simulink model "CompleteAttDetSim"  (R2019b)
settings: Solver=FixedStepAuto  StartTime=0.0  StopTime=24*3600  FixedStep=10  RelTol=1e-3  EnableMultiTasking=on
PreLoadFcn:
  | InitialiseJ2
undefined symbols (not defined in the file): a, e, Earth, h, i, J2, mu, omega, R_earth, RAAN, T, t0, WGS84
libraries: vrlib x11, sharedtransform x9, aerolibutil x5, dspindex x1, aerolibtransform2 x1
settings Model: PauseTimes=0  NumberOfSteps=10  SnapshotBufferSize=10000  SnapshotInterval=1  Creator="TEAM  STUDSAT -2"  LastModifiedBy=zackm
settings DataIOCC: ReturnWorkspaceOutputs=off
settings OptimizationCC: LifeSpan=inf
settings DebuggingCC: SFUnexpectedBacktrackingDiag=warning  SFNoUnconditionalDefaultTransitionDiag=warning  SFExecutionAtInitializationDiag=none  ArithmeticOperatorsInVariantConditions=warning
settings SFSimCC: SimUseLocalCustomCode=off  CustomCodeUndefinedFunction=UseInterfaceOnly
settings RTWCC: RTWUseLocalCustomCode=off
settings CodeAppCC: StateflowObjectComments=on
settings GRTTargetCC: TargetLangStandard=C89/C90 (ANSI)  GeneratePreprocessorConditionals=Disable all
settings ConfigComp: CovMetricSettings=dw  CovHtmlReporting=on  CovSaveCumulativeToWorkspaceVar=on  CovSaveSingleToWorkspaceVar=on  CovExternalEMLEnable=off

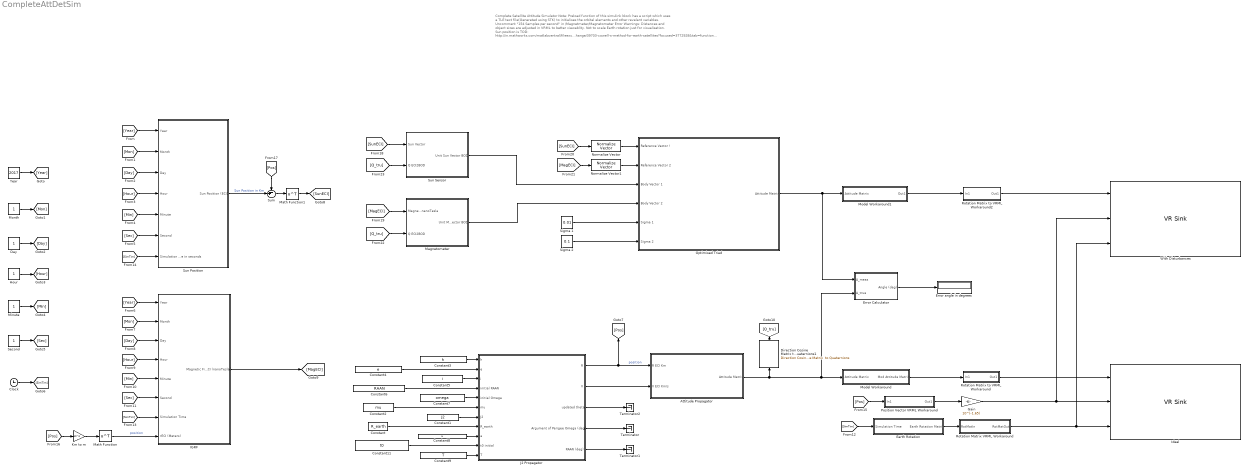
== system CompleteAttDetSim ==
  note: Complete Satellite Attitude Simulator
      |
      | Note:
      | Preload function of this simulink block has a script which uses a TLE text file(Generated using STK) to initialises the orbital elements and other revelant variables.
      | Uncomment "154 Samples per second" in /Magnetmeter/Magnetometer Error
      |
      | Warnings:
      | Distances and object sizes are adjusted in VRML to better viewablity. Not to scale
      | Earth rotation just for visualisation.
      | Sun position is TOD: http://in.mathworks.com/matlabcentral/fileexchange/39703-cowell-s-method-for-earth-satellites?focused=3772928&tab=function
      | Magnetometer model needs improvements
  " Magnetometer" : Subsystem
  " Sun Position" : Subsystem
  Attitude Propagator : Subsystem
  Clock : Clock
  Constant : Constant  Value=R_earth
  Constant1 : Constant  Value=J2
  Constant11 : Constant  Value=t0
  Constant2 : Constant  Value=mu
  Constant3 : Constant  Value=h
  Constant4 : Constant  Value=e
  Constant5 : Constant  Value=i
  Constant6 : Constant  Value=RAAN
  Constant7 : Constant  Value=omega
  Constant8 : Constant  Value=a
  Constant9 : Constant  Value=T
  Day : Constant
  Direction Cosine Matrix to Quaternions1 : sharedtransform/Direction Cosine Matrix  to Quaternions  aMode=aMode  action=None  tolerance=eps(2)
      settings: SourceProductName=Aerospace Blockset  SourceProductBaseCode=AE
  Earth Rotation : Subsystem
  Error Calculator : Subsystem
  Error angle in degrees : Display
  Gain : Gain  Gain=10^(-1.65)
  Hour : Constant
  IGRF : Subsystem
  Ideal : vrlib/VR Sink  InstantiateOnLoad=on  SampleTime=-1  ViewEnable=on  RemoteChange=off  RemoteView=off  FieldsWritten=Satellite.rotation.4.1.1.double#Satellite.translation.3.1.1.double#Earth.rotation.4.1.1.double  WorldFileName=earthSatSys_Ideal.WRL  AutoView=off  VideoDimensions=[]  AllowVariableSize=off
      settings: SourceProductBaseCode=VR
  J2 Propagator : Subsystem
  Km to m : Gain  Gain=10^3
  Math Function : Math  Operator=transpose  SaturateOnIntegerOverflow=on
  Math Function1 : Math  Operator=transpose  SaturateOnIntegerOverflow=on
  Minute : Constant
  Model Workaround : Subsystem
  Model Workaround1 : Subsystem
  Month : Constant
  Normalize Vector : vrlib/Utilities/Normalize Vector  maxzero=0
      settings: SourceProductName=Simulink 3D Animation  SourceProductBaseCode=VR
  Normalize Vector1 : vrlib/Utilities/Normalize Vector  maxzero=0
      settings: SourceProductName=Simulink 3D Animation  SourceProductBaseCode=VR
  Optimised Triad : Subsystem
  Position Vector VRML Workaround : Subsystem
  Rotation Matrix VRML Workaround : Subsystem
  Rotation Matrix to VRML Workaround : Subsystem
  Rotation Matrix to VRML Workaround2 : Subsystem
  Second : Constant
  Sigma 1 : Constant  Value=0.01
  Sigma 2 : Constant  Value=0.1
  Sum : Sum  Inputs=-+|
  Sun Sensor : Subsystem
  Terminator : Terminator
  Terminator1 : Terminator
  Terminator2 : Terminator
  With Disturbances : vrlib/VR Sink  InstantiateOnLoad=on  SampleTime=-1  ViewEnable=on  RemoteChange=off  RemoteView=off  FieldsWritten=Satellite1.rotation.4.1.1.double#Satellite1.translation.3.1.1.double#Earth1.rotation.4.1.1.double  WorldFileName=earthSatSys_Real.WRL  AutoView=off  VideoDimensions=[]  AllowVariableSize=off
      settings: SourceProductBaseCode=VR
  Year : Constant  Value=2017
  wires:
  Constant/1 -> J2 Propagator/8(R_earth)
  Constant1/1 -> J2 Propagator/7(J2)
  Constant2/1 -> J2 Propagator/6(mu)
  Constant3/1 -> J2 Propagator/1(h)
  Constant4/1 -> J2 Propagator/2(e)
  Constant5/1 -> J2 Propagator/3(i)
  Constant6/1 -> J2 Propagator/4(initial RAAN)
  Constant8/1 -> J2 Propagator/9(a)
  Constant11/1 -> J2 Propagator/10(t0 initial)
  Constant9/1 -> J2 Propagator/11(T)
  Constant7/1 -> J2 Propagator/5(initial Omega)
  J2 Propagator/4(Argument of Perigee Omega (deg)) -> Terminator/1
  Earth Rotation/1(Earth Rotation Matrix) -> Rotation Matrix VRML Workaround/1(RotMatIn)
  Position Vector VRML Workaround/1(Out1) -> Gain/1
  J2 Propagator/5(RAAN (deg)) -> Terminator1/1
  Gain/1 -> With Disturbances/2, Ideal/2
  Rotation Matrix VRML Workaround/1(RotMatOut) -> With Disturbances/3, Ideal/3
  J2 Propagator/3(updated theta) -> Terminator2/1
  Model Workaround/1(Mod Attitude Matrix) -> Rotation Matrix to VRML Workaround/1(In1)
  J2 Propagator/2(V) -> Attitude Propagator/2(V ECI Km/s)
  Rotation Matrix to VRML Workaround/1(Out1) -> Ideal/1
  Model Workaround1/1(Out1) -> Rotation Matrix to VRML Workaround2/1(In1)
  Sigma 2/1 -> Optimised Triad/6(Sigma 2)
  Optimised Triad/1(Attitude Matrix) -> Error Calculator/1(A_meas), Model Workaround1/1(Attitude Matrix)
  Rotation Matrix to VRML Workaround2/1(Out1) -> With Disturbances/1
  Sigma 1/1 -> Optimised Triad/5(Sigma 1)
  " Magnetometer"/1(Unit Magnetic Field Vector BOD) -> Optimised Triad/4(Body Vector 2)
  Error Calculator/1(Angle (deg)) -> Error angle in degrees/1
  Km to m/1 -> Math Function/1
  " Sun Position"/1(Sun Position (ECI)) -> Sum/2  "Sun Position in Km"
  Attitude Propagator/1(Attitude Matrix) -> Direction Cosine Matrix to Quaternions1/1, Error Calculator/2(A_true), Model Workaround/1(Attitude Matrix)
  Sun Sensor/1(Unit Sun Vector BOD) -> Optimised Triad/3(Body Vector 1)
  Year/1 -> [Year]
  Month/1 -> [Mon]
  Day/1 -> [Day]
  Hour/1 -> [Hour]
  Minute/1 -> [Min]
  Second/1 -> [Sec]
  [Year] -> " Sun Position"/1(Year)
  [Mon] -> " Sun Position"/2("Month ")
  [Day] -> " Sun Position"/3(Day)
  [Hour] -> " Sun Position"/4(Hour)
  [Min] -> " Sun Position"/5(Minute)
  [Sec] -> " Sun Position"/6(Second)
  [Year] -> IGRF/1(Year)
  [Mon] -> IGRF/2(Month)
  [Day] -> IGRF/3(Day)
  [Hour] -> IGRF/4(Hour)
  [Min] -> IGRF/5(Minute)
  [Sec] -> IGRF/6(Second)
  Clock/1 -> [SimTim]
  [SimTim] -> Earth Rotation/1(Simulation Time)
  [SimTim] -> IGRF/7(Simulation Time)
  [SimTim] -> " Sun Position"/7(" Simulation time in seconds")
  J2 Propagator/1(R) -> [Pos], Attitude Propagator/1(R ECI Km)  "position"
  [Pos] -> Position Vector VRML Workaround/1(In1)
  [Pos] -> Km to m/1
  Math Function/1 -> IGRF/8(rECI (Meters))  "position"
  [Pos] -> Sum/1
  Sum/1 -> Math Function1/1
  IGRF/1(Magnetic Field in ECI (nanoTesla)) -> [MagECI]
  [SunECI] -> Sun Sensor/1(Sun Vector)
  [MagECI] -> " Magnetometer"/1(Magnettic Field ECI nanoTesla)
  [SunECI] -> Normalize Vector/1
  [MagECI] -> Normalize Vector1/1
  Normalize Vector/1 -> Optimised Triad/1(Reference Vector !)
  Normalize Vector1/1 -> Optimised Triad/2(Reference Vector 2)
  Direction Cosine Matrix to Quaternions1/1 -> [Q_tru]
  [Q_tru] -> " Magnetometer"/2(Q ECI2BOD)
  [Q_tru] -> Sun Sensor/2(Q ECI2BOD)
  Math Function1/1 -> [SunECI]

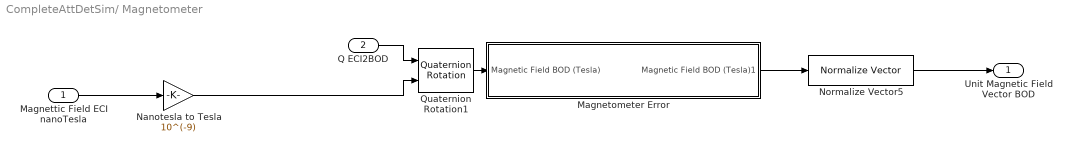
== system CompleteAttDetSim/ Magnetometer ==
  Magnettic Field ECI nanoTesla : Inport
  Q ECI2BOD : Inport  Port=2
  Magnetometer Error : Subsystem
  Nanotesla to Tesla : Gain  Gain=10^(-9)
  Normalize Vector5 : vrlib/Utilities/Normalize Vector  maxzero=0
      settings: SourceProductName=Simulink 3D Animation  SourceProductBaseCode=VR
  Quaternion Rotation1 : aerolibutil/Quaternion Rotation
  Unit Magnetic Field Vector BOD : Outport
  wires:
  Magnettic Field ECI nanoTesla/1 -> Nanotesla to Tesla/1
  Magnetometer Error/1("Magnetic Field BOD (Tesla)1 ") -> Normalize Vector5/1
  Normalize Vector5/1 -> Unit Magnetic Field Vector BOD/1
  Q ECI2BOD/1 -> Quaternion Rotation1/1
  Nanotesla to Tesla/1 -> Quaternion Rotation1/2
  Quaternion Rotation1/1 -> Magnetometer Error/1(Magnetic Field BOD (Tesla))

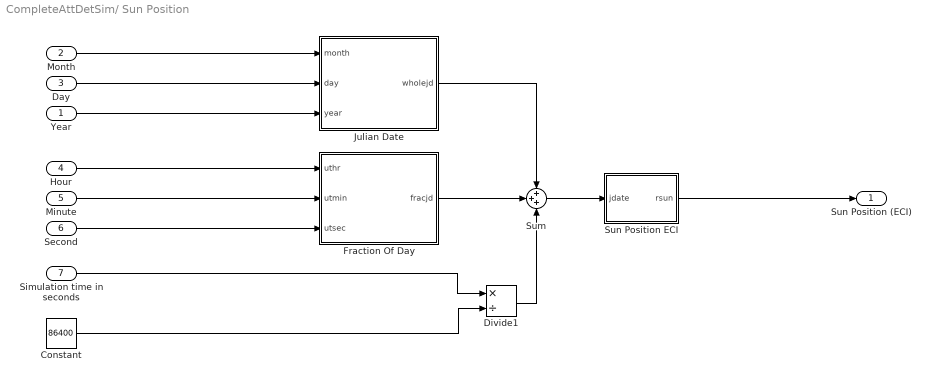
== system CompleteAttDetSim/ Sun Position ==
  Year : Inport
  "Month " : Inport  Port=2
  Day : Inport  Port=3
  Hour : Inport  Port=4
  Minute : Inport  Port=5
  Second : Inport  Port=6
  " Simulation time in seconds" : Inport  Port=7
  Constant : Constant  Value=86400
  Divide1 : Product  Inputs=*/
  Fraction Of Day : MATLAB Function  TreatAsAtomicUnit=on
  Julian Date : MATLAB Function  TreatAsAtomicUnit=on
  Sum : Sum  Inputs=+++
  Sun Position ECI : MATLAB Function  TreatAsAtomicUnit=on
  Sun Position (ECI) : Outport
  wires:
  Sum/1 -> Sun Position ECI/1(jdate)
  " Simulation time in seconds"/1 -> Divide1/1
  Sun Position ECI/1(rsun) -> Sun Position (ECI)/1
  Second/1 -> Fraction Of Day/3(utsec)
  Fraction Of Day/1(fracjd) -> Sum/2
  Year/1 -> Julian Date/3(year)
  Day/1 -> Julian Date/2(day)
  Divide1/1 -> Sum/3
  Minute/1 -> Fraction Of Day/2(utmin)
  Julian Date/1(wholejd) -> Sum/1
  Constant/1 -> Divide1/2
  Hour/1 -> Fraction Of Day/1(uthr)
  "Month "/1 -> Julian Date/1(month)

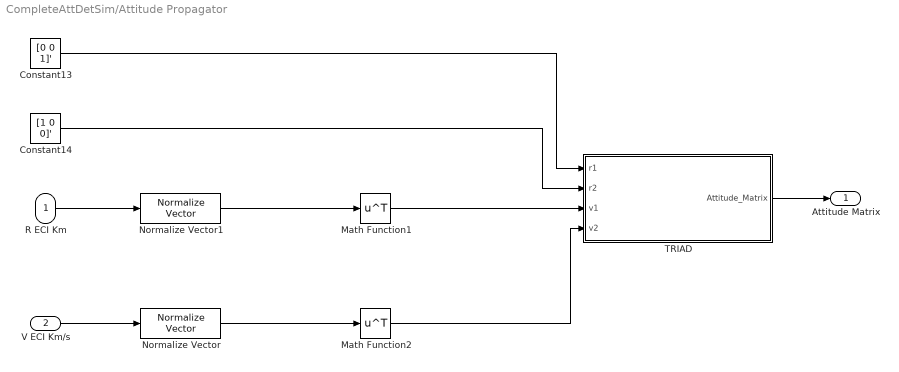
== system CompleteAttDetSim/Attitude Propagator ==
  R ECI Km : Inport
  V ECI Km/s : Inport  Port=2
  Constant13 : Constant  Value=[0 0 1]'  VectorParams1D=off
  Constant14 : Constant  Value=[1 0 0]'  VectorParams1D=off
  Math Function1 : Math  Operator=transpose  SaturateOnIntegerOverflow=on
  Math Function2 : Math  Operator=transpose  SaturateOnIntegerOverflow=on
  Normalize Vector : vrlib/Utilities/Normalize Vector  maxzero=0
      settings: SourceProductName=Simulink 3D Animation  SourceProductBaseCode=VR
  Normalize Vector1 : vrlib/Utilities/Normalize Vector  maxzero=0
      settings: SourceProductName=Simulink 3D Animation  SourceProductBaseCode=VR
  TRIAD : MATLAB Function  TreatAsAtomicUnit=on
  Attitude Matrix : Outport
  wires:
  Constant13/1 -> TRIAD/1(r1)
  TRIAD/1(Attitude_Matrix) -> Attitude Matrix/1
  Math Function1/1 -> TRIAD/3(v1)
  Math Function2/1 -> TRIAD/4(v2)
  Constant14/1 -> TRIAD/2(r2)
  V ECI Km/s/1 -> Normalize Vector/1
  Normalize Vector/1 -> Math Function2/1
  Normalize Vector1/1 -> Math Function1/1
  R ECI Km/1 -> Normalize Vector1/1

== system CompleteAttDetSim/Earth Rotation ==
  Simulation Time : Inport
  Constant10 : Constant  Value=0.004178074378280
  Subsystem1 : Subsystem
  Earth Rotation Matrix : Outport
  wires:
  Constant10/1 -> Subsystem1/1(we)
  Simulation Time/1 -> Subsystem1/2(Clock)
  Subsystem1/1(Earth Rotation Matrix) -> Earth Rotation Matrix/1

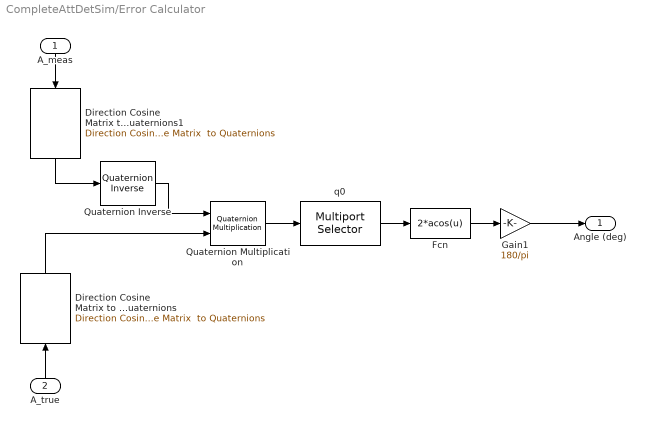
== system CompleteAttDetSim/Error Calculator ==
  A_meas : Inport
  A_true : Inport  Port=2
  Direction Cosine Matrix to Quaternions : sharedtransform/Direction Cosine Matrix  to Quaternions  aMode=aMode  action=None  tolerance=eps(2)
      settings: SourceProductName=Aerospace Blockset  SourceProductBaseCode=AE
  Direction Cosine Matrix to Quaternions1 : sharedtransform/Direction Cosine Matrix  to Quaternions  aMode=aMode  action=None  tolerance=eps(2)
      settings: SourceProductName=Aerospace Blockset  SourceProductBaseCode=AE
  Fcn : Fcn  Expr=2*acos(u)
  Gain1 : Gain  Gain=180/pi
  Quaternion Inverse : aerolibutil/Quaternion Inverse
      settings: SourceProductName=Aerospace Blockset
  Quaternion Multiplication : aerolibutil/Quaternion Multiplication
  q0 : dspindex/Multiport Selector  rowsOrCols=Rows  idxCellArray={ 1 }  idxErrMode=Clip Index
  Angle (deg) : Outport
  wires:
  q0/1 -> Fcn/1
  Fcn/1 -> Gain1/1
  Gain1/1 -> Angle (deg)/1
  Direction Cosine Matrix to Quaternions1/1 -> Quaternion Inverse/1
  A_meas/1 -> Direction Cosine Matrix to Quaternions1/1
  A_true/1 -> Direction Cosine Matrix to Quaternions/1
  Quaternion Inverse/1 -> Quaternion Multiplication/1
  Quaternion Multiplication/1 -> q0/1
  Direction Cosine Matrix to Quaternions/1 -> Quaternion Multiplication/2

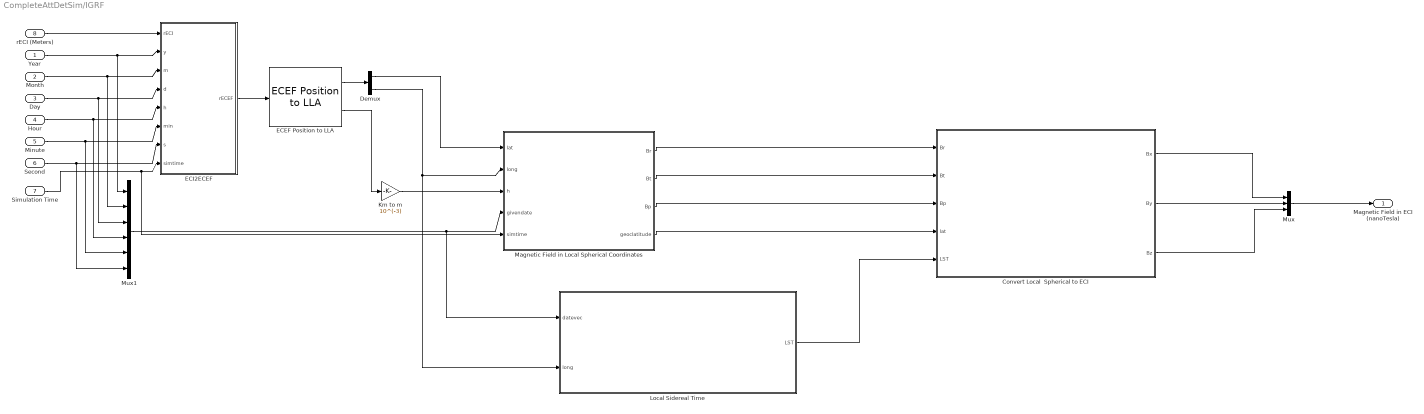
== system CompleteAttDetSim/IGRF ==
  Year : Inport
  Month : Inport  Port=2
  Day : Inport  Port=3
  Hour : Inport  Port=4
  Minute : Inport  Port=5
  Second : Inport  Port=6
  Simulation Time : Inport  Port=7
  rECI (Meters) : Inport  Port=8
  Convert Local  Spherical to ECI : MATLAB Function  TreatAsAtomicUnit=on
  Demux : Demux  Outputs=2
  ECEF Position to LLA : aerolibtransform2/ECEF Position to LLA  units=Metric (MKS)  ptype=Earth (WGS84)  F=1/298.257223563  R=6378137
      settings: SourceProductName=Aerospace Blockset  SourceProductBaseCode=AE
  ECI2ECEF : MATLAB Function  TreatAsAtomicUnit=on
  Km to m : Gain  Gain=10^(-3)
  Local Sidereal Time : MATLAB Function  TreatAsAtomicUnit=on
  Magnetic Field in Local Spherical Coordinates : MATLAB Function  TreatAsAtomicUnit=on
  Mux : Mux  Inputs=3
  Mux1 : Mux  Inputs=6
  Magnetic Field in ECI (nanoTesla) : Outport
  wires:
  Magnetic Field in Local Spherical Coordinates/2(Bt) -> Convert Local  Spherical to ECI/2(Bt)
  Day/1 -> Mux1/3, ECI2ECEF/4(d)
  Second/1 -> Mux1/6, ECI2ECEF/7(s)
  ECEF Position to LLA/1 -> Demux/1
  Convert Local  Spherical to ECI/3(Bz) -> Mux/3
  Magnetic Field in Local Spherical Coordinates/3(Bp) -> Convert Local  Spherical to ECI/3(Bp)
  Local Sidereal Time/1(LST) -> Convert Local  Spherical to ECI/5(LST)
  Magnetic Field in Local Spherical Coordinates/1(Br) -> Convert Local  Spherical to ECI/1(Br)
  ECEF Position to LLA/2 -> Km to m/1
  Minute/1 -> Mux1/5, ECI2ECEF/6(min)
  ECI2ECEF/1(rECEF) -> ECEF Position to LLA/1
  Demux/1 -> Magnetic Field in Local Spherical Coordinates/1(lat)
  Month/1 -> Mux1/2, ECI2ECEF/3(m)
  Year/1 -> Mux1/1, ECI2ECEF/2(y)
  rECI (Meters)/1 -> ECI2ECEF/1(rECI)
  Convert Local  Spherical to ECI/1(Bx) -> Mux/1
  Magnetic Field in Local Spherical Coordinates/4(geoclatitude) -> Convert Local  Spherical to ECI/4(lat)
  Hour/1 -> Mux1/4, ECI2ECEF/5(h)
  Mux1/1 -> Magnetic Field in Local Spherical Coordinates/4(givendate), Local Sidereal Time/1(datevec)
  Convert Local  Spherical to ECI/2(By) -> Mux/2
  Demux/2 -> Local Sidereal Time/2(long), Magnetic Field in Local Spherical Coordinates/2(long)
  Mux/1 -> Magnetic Field in ECI (nanoTesla)/1
  Simulation Time/1 -> ECI2ECEF/8(simtime), Magnetic Field in Local Spherical Coordinates/5(simtime)
  Km to m/1 -> Magnetic Field in Local Spherical Coordinates/3(h)

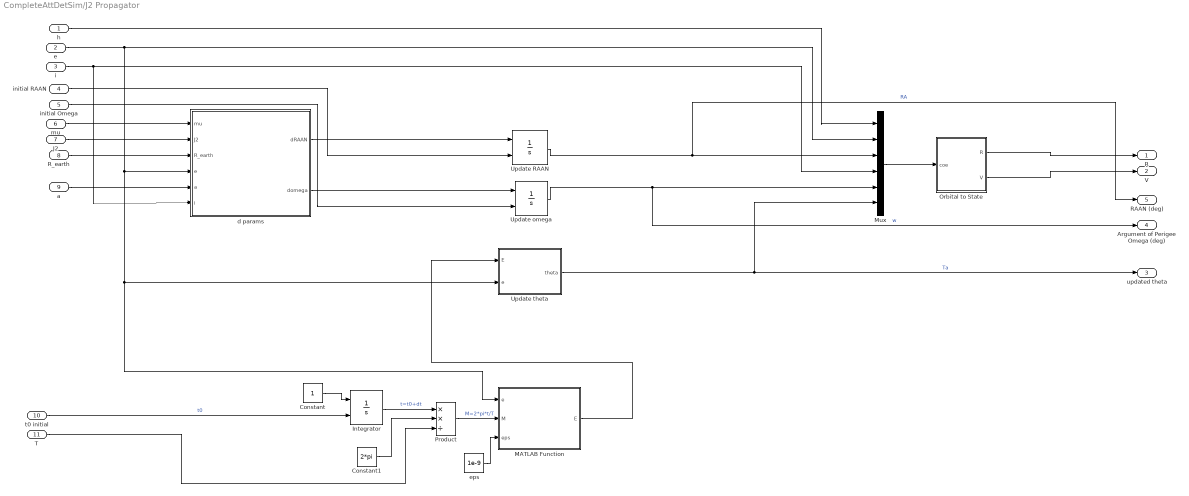
== system CompleteAttDetSim/J2 Propagator ==
  h : Inport
  e : Inport  Port=2
  i : Inport  Port=3
  initial RAAN : Inport  Port=4
  initial Omega : Inport  Port=5
  mu : Inport  Port=6
  J2 : Inport  Port=7
  R_earth : Inport  Port=8
  a : Inport  Port=9
  t0 initial : Inport  Port=10
  T : Inport  Port=11
  Constant : Constant
  Constant1 : Constant  Value=2*pi
  Integrator : Integrator  InitialConditionSource=external
  MATLAB Function : MATLAB Function  TreatAsAtomicUnit=on
  Mux : Mux  Inputs=6
  Orbital to State : MATLAB Function  TreatAsAtomicUnit=on
  Product : Product  Inputs=**/
  Update RAAN : Integrator  InitialConditionSource=external
  Update omega : Integrator  InitialConditionSource=external
  Update theta : MATLAB Function  TreatAsAtomicUnit=on
  d params : MATLAB Function  TreatAsAtomicUnit=on
  eps : Constant  Value=1e-9
  R : Outport
  V : Outport  Port=2
  updated theta : Outport  Port=3
  Argument of Perigee Omega (deg) : Outport  Port=4
  RAAN (deg) : Outport  Port=5
  wires:
  eps/1 -> MATLAB Function/3(eps)
  mu/1 -> d params/1(mu)
  a/1 -> d params/5(a)
  J2/1 -> d params/2(J2)
  R_earth/1 -> d params/3(R_earth)
  MATLAB Function/1(E) -> Update theta/1(E)
  t0 initial/1 -> Integrator/2  "t0"
  Constant/1 -> Integrator/1
  Integrator/1 -> Product/1  "t=t0+dt"
  T/1 -> Product/3
  Constant1/1 -> Product/2
  d params/1(dRAAN) -> Update RAAN/1
  initial RAAN/1 -> Update RAAN/2
  d params/2(domega) -> Update omega/1
  initial Omega/1 -> Update omega/2
  h/1 -> Mux/1
  i/1 -> d params/6(i), Mux/4
  Mux/1 -> Orbital to State/1(coe)
  Product/1 -> MATLAB Function/2(M)  "M=2*pi*t/T"
  Update omega/1 -> Argument of Perigee Omega (deg)/1, Mux/5  "w"
  Update theta/1(theta) -> Mux/6, updated theta/1  "Ta"
  Update RAAN/1 -> RAAN (deg)/1, Mux/3  "RA"
  e/1 -> MATLAB Function/1(e), Update theta/2(e), d params/4(e), Mux/2
  Orbital to State/1(R) -> R/1
  Orbital to State/2(V) -> V/1

== system CompleteAttDetSim/Model Workaround ==
  Attitude Matrix : Inport
  Constant10 : Constant  Value=-90
  Matrix Multiply1 : Product  Multiplication=Matrix(*)
  Rotate about x1 : MATLAB Function  TreatAsAtomicUnit=on
  Mod Attitude Matrix : Outport
  wires:
  Constant10/1 -> Rotate about x1/1(u)
  Matrix Multiply1/1 -> Mod Attitude Matrix/1
  Attitude Matrix/1 -> Matrix Multiply1/1
  Rotate about x1/1(y) -> Matrix Multiply1/2

== system CompleteAttDetSim/Model Workaround1 ==
  Attitude Matrix : Inport
  Constant10 : Constant  Value=-90
  Matrix Multiply1 : Product  Multiplication=Matrix(*)
  Rotate about x1 : MATLAB Function  TreatAsAtomicUnit=on
  Out1 : Outport
  wires:
  Constant10/1 -> Rotate about x1/1(u)
  Matrix Multiply1/1 -> Out1/1
  Attitude Matrix/1 -> Matrix Multiply1/1
  Rotate about x1/1(y) -> Matrix Multiply1/2

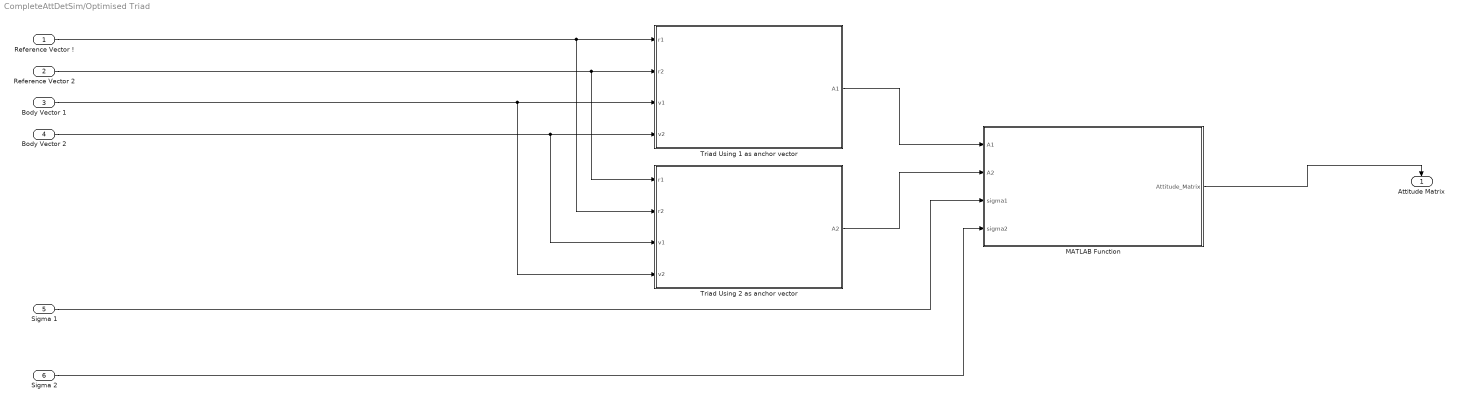
== system CompleteAttDetSim/Optimised Triad ==
  Reference Vector ! : Inport
  Reference Vector 2 : Inport  Port=2
  Body Vector 1 : Inport  Port=3
  Body Vector 2 : Inport  Port=4
  Sigma 1 : Inport  Port=5
  Sigma 2 : Inport  Port=6
  MATLAB Function : MATLAB Function  TreatAsAtomicUnit=on
  Triad Using 1 as anchor vector : MATLAB Function  TreatAsAtomicUnit=on
  Triad Using 2 as anchor vector : MATLAB Function  TreatAsAtomicUnit=on
  Attitude Matrix : Outport
  wires:
  Triad Using 1 as anchor vector/1(A1) -> MATLAB Function/1(A1)
  Sigma 2/1 -> MATLAB Function/4(sigma2)
  Body Vector 2/1 -> Triad Using 1 as anchor vector/4(v2), Triad Using 2 as anchor vector/3(v1)
  Body Vector 1/1 -> Triad Using 2 as anchor vector/4(v2), Triad Using 1 as anchor vector/3(v1)
  Sigma 1/1 -> MATLAB Function/3(sigma1)
  Triad Using 2 as anchor vector/1(A2) -> MATLAB Function/2(A2)
  Reference Vector 2/1 -> Triad Using 1 as anchor vector/2(r2), Triad Using 2 as anchor vector/1(r1)
  MATLAB Function/1(Attitude_Matrix) -> Attitude Matrix/1
  Reference Vector !/1 -> Triad Using 2 as anchor vector/2(r2), Triad Using 1 as anchor vector/1(r1)

== system CompleteAttDetSim/Position Vector VRML Workaround ==
  In1 : Inport
  Demux : Demux  Outputs=3
  Gain2 : Gain  Gain=-1
  Mux : Mux  Inputs=3
  Out1 : Outport
  wires:
  Demux/1 -> Mux/1
  Demux/2 -> Gain2/1
  Demux/3 -> Mux/2
  Mux/1 -> Out1/1
  Gain2/1 -> Mux/3
  In1/1 -> Demux/1

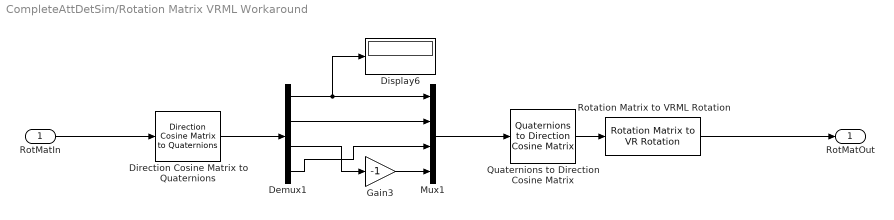
== system CompleteAttDetSim/Rotation Matrix VRML Workaround ==
  RotMatIn : Inport
  Demux1 : Demux
  Direction Cosine Matrix to Quaternions : sharedtransform/Direction Cosine Matrix  to Quaternions  aMode=aMode  action=None  tolerance=eps(2)
      settings: SourceProductName=Aerospace Blockset  SourceProductBaseCode=AE
  Display6 : Display
  Gain3 : Gain  Gain=-1
  Mux1 : Mux
  Quaternions to Direction Cosine Matrix : sharedtransform/Quaternions to  Direction Cosine Matrix  aMode=aMode
      settings: SourceProductName=Aerospace Blockset  SourceProductBaseCode=AE
  Rotation Matrix to VRML Rotation : vrlib/Utilities/Rotation Matrix to VR Rotation  maxzero=1e-12
      settings: SourceProductName=Simulink 3D Animation  SourceProductBaseCode=VR
  RotMatOut : Outport
  wires:
  RotMatIn/1 -> Direction Cosine Matrix to Quaternions/1
  Direction Cosine Matrix to Quaternions/1 -> Demux1/1
  Demux1/3 -> Gain3/1
  Gain3/1 -> Mux1/4
  Demux1/4 -> Mux1/3
  Demux1/2 -> Mux1/2
  Demux1/1 -> Display6/1, Mux1/1
  Mux1/1 -> Quaternions to Direction Cosine Matrix/1
  Quaternions to Direction Cosine Matrix/1 -> Rotation Matrix to VRML Rotation/1
  Rotation Matrix to VRML Rotation/1 -> RotMatOut/1

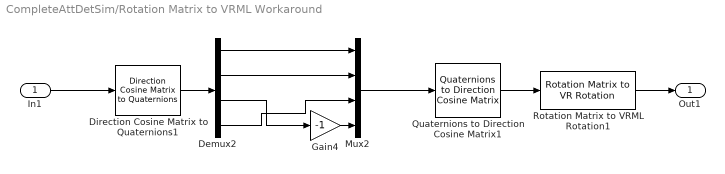
== system CompleteAttDetSim/Rotation Matrix to VRML Workaround ==
  In1 : Inport
  Demux2 : Demux
  Direction Cosine Matrix to Quaternions1 : sharedtransform/Direction Cosine Matrix  to Quaternions  aMode=aMode  action=None  tolerance=eps(2)
      settings: SourceProductName=Aerospace Blockset  SourceProductBaseCode=AE
  Gain4 : Gain  Gain=-1
  Mux2 : Mux
  Quaternions to Direction Cosine Matrix1 : sharedtransform/Quaternions to  Direction Cosine Matrix  aMode=aMode
      settings: SourceProductName=Aerospace Blockset  SourceProductBaseCode=AE
  Rotation Matrix to VRML Rotation1 : vrlib/Utilities/Rotation Matrix to VR Rotation  maxzero=1e-12
      settings: SourceProductName=Simulink 3D Animation  SourceProductBaseCode=VR
  Out1 : Outport
  wires:
  Direction Cosine Matrix to Quaternions1/1 -> Demux2/1
  Rotation Matrix to VRML Rotation1/1 -> Out1/1
  Mux2/1 -> Quaternions to Direction Cosine Matrix1/1
  Demux2/4 -> Mux2/3
  Demux2/3 -> Gain4/1
  Gain4/1 -> Mux2/4
  Demux2/1 -> Mux2/1
  Demux2/2 -> Mux2/2
  Quaternions to Direction Cosine Matrix1/1 -> Rotation Matrix to VRML Rotation1/1
  In1/1 -> Direction Cosine Matrix to Quaternions1/1

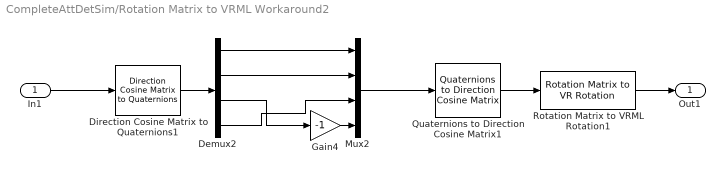
== system CompleteAttDetSim/Rotation Matrix to VRML Workaround2 ==
  In1 : Inport
  Demux2 : Demux
  Direction Cosine Matrix to Quaternions1 : sharedtransform/Direction Cosine Matrix  to Quaternions  aMode=aMode  action=None  tolerance=eps(2)
      settings: SourceProductName=Aerospace Blockset  SourceProductBaseCode=AE
  Gain4 : Gain  Gain=-1
  Mux2 : Mux
  Quaternions to Direction Cosine Matrix1 : sharedtransform/Quaternions to  Direction Cosine Matrix  aMode=aMode
      settings: SourceProductName=Aerospace Blockset  SourceProductBaseCode=AE
  Rotation Matrix to VRML Rotation1 : vrlib/Utilities/Rotation Matrix to VR Rotation  maxzero=1e-12
      settings: SourceProductName=Simulink 3D Animation  SourceProductBaseCode=VR
  Out1 : Outport
  wires:
  Direction Cosine Matrix to Quaternions1/1 -> Demux2/1
  Rotation Matrix to VRML Rotation1/1 -> Out1/1
  Mux2/1 -> Quaternions to Direction Cosine Matrix1/1
  Demux2/4 -> Mux2/3
  Demux2/3 -> Gain4/1
  Gain4/1 -> Mux2/4
  Demux2/1 -> Mux2/1
  Demux2/2 -> Mux2/2
  Quaternions to Direction Cosine Matrix1/1 -> Rotation Matrix to VRML Rotation1/1
  In1/1 -> Direction Cosine Matrix to Quaternions1/1

== system CompleteAttDetSim/Sun Sensor ==
  Sun Vector : Inport
  Q ECI2BOD : Inport  Port=2
  MATLAB Function : MATLAB Function  TreatAsAtomicUnit=on
  Normalize Vector4 : vrlib/Utilities/Normalize Vector  maxzero=0
      settings: SourceProductName=Simulink 3D Animation  SourceProductBaseCode=VR
  Quaternion Rotation : aerolibutil/Quaternion Rotation
  Quaternion Rotation2 : aerolibutil/Quaternion Rotation
  Unit Sun Vector BOD : Outport
  wires:
  Sun Vector/1 -> Quaternion Rotation/2
  MATLAB Function/1(quat) -> Quaternion Rotation/1
  Normalize Vector4/1 -> Unit Sun Vector BOD/1
  Q ECI2BOD/1 -> Quaternion Rotation2/1
  Quaternion Rotation2/1 -> Normalize Vector4/1
  Quaternion Rotation/1 -> Quaternion Rotation2/2

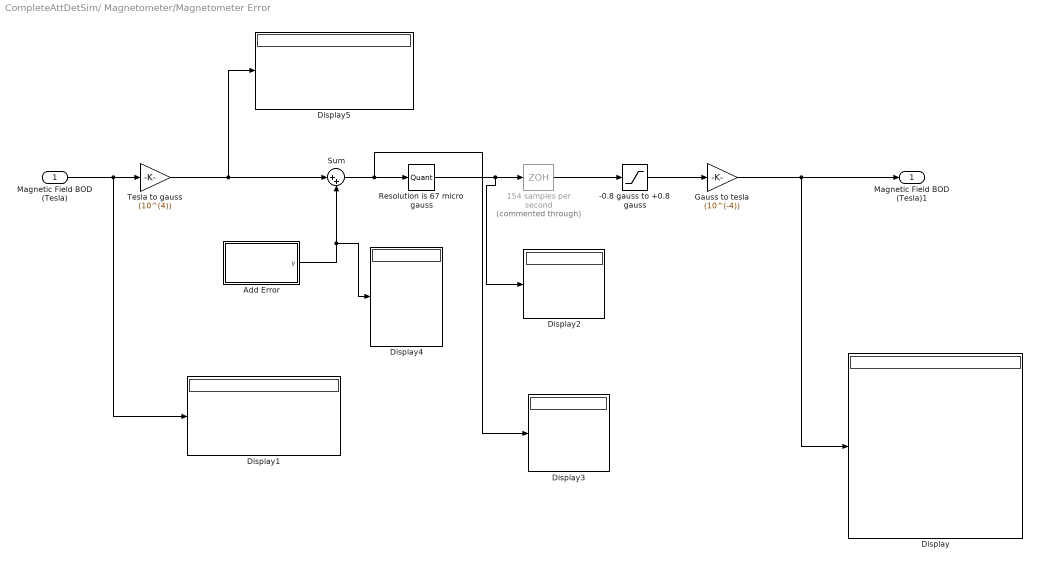
== system CompleteAttDetSim/ Magnetometer/Magnetometer Error ==
  Magnetic Field BOD (Tesla) : Inport
  -0.8 gauss to +0.8 gauss : Saturate  UpperLimit=0.8  LowerLimit=-0.8
  154 samples per second : ZeroOrderHold  Commented=through  SampleTime=1/154
  Add Error : MATLAB Function  TreatAsAtomicUnit=on
  Display{,1..5} (6 alike) : Display
  Gauss to tesla : Gain  Gain=(10^(-4))
  Resolution is 67 micro gauss : Quantizer  QuantizationInterval=67*10^(-3)
  Sum : Sum  Inputs=|++
  Tesla to gauss : Gain  Gain=(10^(4))
  "Magnetic Field BOD (Tesla)1 " : Outport
  wires:
  -0.8 gauss to +0.8 gauss/1 -> Gauss to tesla/1
  Sum/1 -> Display3/1, Resolution is 67 micro gauss/1
  Resolution is 67 micro gauss/1 -> Display2/1, 154 samples per second/1
  Tesla to gauss/1 -> Display5/1, Sum/1
  Add Error/1(y) -> Display4/1, Sum/2
  154 samples per second/1 -> -0.8 gauss to +0.8 gauss/1
  Magnetic Field BOD (Tesla)/1 -> Display1/1, Tesla to gauss/1
  Gauss to tesla/1 -> Display/1, "Magnetic Field BOD (Tesla)1 "/1

== system CompleteAttDetSim/Earth Rotation/Subsystem1 ==
  we : Inport
  Clock : Inport  Port=2
  Display : Display
  MATLAB Function : MATLAB Function  TreatAsAtomicUnit=on
  Product1 : Product
  Earth Rotation Matrix : Outport
  wires:
  Clock/1 -> Product1/2
  we/1 -> Product1/1
  Product1/1 -> MATLAB Function/1(u), Display/1  "fi_earth"
  MATLAB Function/1(y) -> Earth Rotation Matrix/1

== matlab function CompleteAttDetSim/Earth Rotation/Subsystem1/MATLAB Function ==
  data: u input; y output
function y = fcn(u)
%#codegen

y =rotz(u);

== matlab function CompleteAttDetSim/J2 Propagator/d params ==
  data: mu input; dRAAN output; J2 input; R_earth input; e input; a input; i input; domega output
function [dRAAN, domega]=dparams(mu,J2, R_earth,e,a,i)

dRAAN = -(1.5*mu^0.5*J2*R_earth^2/((1-e^2)*a^3.5))*cosd(i)*180/pi;
domega = dRAAN*(2.5*sind(i)^2 - 2)/cosd(i);
end

== matlab function CompleteAttDetSim/Model Workaround1/Rotate about x1 ==
  data: u input; y output
function y = fcn(u)
%#codegen

y =rotx(u);

== matlab function CompleteAttDetSim/J2 Propagator/MATLAB Function ==
  data: e input; M input; E output; eps input
function E = keplerEq(e,M,eps)
En  = M;
Ens = En - (En-e*sin(En)- M)/(1 - e*cos(En));
while ( abs(Ens-En) > eps )
    En = Ens;
    Ens = En - (En - e*sin(En) - M)/(1 - e*cos(En));
end;
E = Ens;
end

== matlab function CompleteAttDetSim/J2 Propagator/Update theta ==
  data: E input; theta output; e input
function theta = updateTheta(E,e)
theta=2*atan(tan(E/2)*((1+e)/(1-e))^0.5)*180/pi;

end

== matlab function CompleteAttDetSim/J2 Propagator/Orbital to State ==
  data: coe input; R output size=[1 3]; V output size=[1 3]
function [R, V] = Orbital2State(coe)

% ˜˜˜˜˜˜˜˜˜˜˜˜˜˜˜˜˜˜˜˜˜˜˜˜˜˜˜˜˜˜˜˜˜˜
% This function computes the state vector (r,v) from the
% classical orbital elements (coe).
%
% mu - gravitational parameter (kmˆ3; sˆ2)
% coe - orbital elements [h e RA incl w TA]
% where
% h = angular momentum (kmˆ2/s)
% e = eccentricity
% RA = right ascension of the ascending node (rad)
% incl = inclination of the orbit (rad)
% w = argument of perigee (rad)
% TA = true anomaly (rad)
% R3_w - Rotation matrix about the z-axis through the angle w
% R1_i - Rotation matrix about the x-axis through the angle i
% R3_W - Rotation matrix about the z-axis through the angle RA
% Q_pX - Matrix of the transformation from perifocal to
% geocentric equatorial frame
% rp - position vector in the perifocal frame (km)
% vp - velocity vector in the perifocal frame (km/s)
% r - position vector in the geocentric equatorial frame
% (km)
% v - velocity vector in the geocentric equatorial frame
% (km/s)
%
% User M-functions required: none
% ------------------------------------------------------------
mu    = 398600; 
h = coe(1);
e = coe(2);
RA = coe(3)*pi/180;
incl = coe(4)*pi/180;
w = coe(5)*pi/180;
TA = coe(6)*pi/180;
%...Equations 4.37 and 4.38 (rp and vp are column vectors):
rp = (h^2/mu) * (1/(1 + e*cos(TA))) * (cos(TA)*[1;0;0] ...
+ sin(TA)*[0;1;0]);
vp = (mu/h) * (-sin(TA)*[1;0;0] + (e + cos(TA))*[0;1;0]);
%...Equation 4.39:
R3_W = [ cos(RA) sin(RA) 0
-sin(RA) cos(RA) 0
0 0 1];
%...Equation 4.40:
R1_i = [1 0 0
0 cos(incl) sin(incl)
0 -sin(incl) cos(incl)];
%...Equation 4.41:
R3_w = [ cos(w) sin(w) 0
-sin(w) cos(w) 0
0 0 1];
%...Equation 4.44:
Q_pX = R3_W'*R1_i'*R3_w';
%...Equations 4.46 (r and v are column vectors):
r = Q_pX*rp;
v = Q_pX*vp;
%...Convert r and v into row vectors:
R = r';
V = v';
% ˜˜˜˜˜˜˜˜˜˜˜˜˜˜˜˜˜˜˜˜˜˜˜˜˜˜˜˜˜˜˜˜˜˜˜˜˜˜˜˜˜˜˜˜˜˜˜˜˜˜˜˜˜˜˜˜˜˜˜˜

== matlab function CompleteAttDetSim/IGRF/Convert Local  Spherical to ECI ==
  data: Br input; Bx output; Bt input; Bp input; lat input; LST input; By output; Bz output
function [Bx,By,Bz] = msph2inert(Br,Bt,Bp,lat, LST)
% Inputs
% Br B in radial direction | Magnetic field strength (B)
% Bt B in theta direction | in local tangential coordinates
% Bp B in phi direction |
% LST Local sidereal time of location (in degrees)
% lat Latitude measured positive north from equator (in degrees)
% Outputs
% Bx B in x-direction | Magnetic field strength (B)
% By B in y-direction | in geocentric inertial coordinates
% Bz B in z-direction |
% Angle conversion to radians
lat=lat*pi/180; LST=LST*pi/180;
% Coordinate transformation
Bx = (Br*cos(lat)+Bt*sin(lat))*cos(LST) - Bp*sin(LST);
By = (Br*cos(lat)+Bt*sin(lat))*sin(LST) + Bp*cos(LST);
Bz = (Br*sin(lat)+Bt*cos(lat));

== matlab function CompleteAttDetSim/IGRF/ECI2ECEF ==
  data: rECI input; rECEF output; y input; m input; d input; h input; min input; s input; simtime input
function rECEF=rECI2ECEF(rECI, y, m, d, h, min, s, simtime )
d2000=367*y-floor((7*(y+(floor(m+9)/12)))/4)+floor(275*m/9)+((h+(min/60)+((s+simtime)/3600))/24)+d-730531.5;
theta=280.46061837+360.98564736628*d2000;

transmat=[cosd(theta) sind(theta) 0;
    -sind(theta) cosd(theta) 0;
    0 0 1];

rECEF=transmat*rECI;

end

== matlab function CompleteAttDetSim/IGRF/Local Sidereal Time ==
  data: datevec input; LST output; long input

function LST = locst(datevec,long)
yr=datevec(1); mon=datevec(2); day=datevec(3); hr=datevec(4); min=datevec(5); sec=datevec(6);
UT=( (sec/60.0 + min ) / 60.0 + hr );
J0 = 367.0 * yr  ...
- floor( (7 * (yr + floor( (mon + 9) / 12.0) ) ) * 0.25 )   ...
+ floor( 275 * mon / 9.0 ) ...
+ day + 1721013.5;
JD=J0+(UT/24);
JC = (J0 - 2451545.0)/36525;
GST0 = 100.4606184 + 36000.77004*JC + 0.000387933*JC^2 - 2.583e-8*JC^3; %[deg]
GST0 = mod(GST0, 360);  % GST0 range [0..360]
GST = GST0 + 360.98564724*UT/24;
GST = mod(GST, 360);  % GST0 range [0..360]
LST = GST + long;
LST = mod(LST, 360);  % LST range [0..360]

== matlab function CompleteAttDetSim/IGRF/Magnetic Field in Local Spherical Coordinates ==
  data: lat input; Br output; long input; h input; givendate input; Bt output; Bp output; geoclatitude output; simtime input

function [Br,Bt,Bp,geoclatitude] = Magfield_Spherical(lat,long,h,givendate, simtime)

%%%%%%%%%%%%%%Calculates Magnetic field in Spherical Coordinates%%%%%%%%%%%

%
% Inputs
% h Geodectic radius (Km)
% lat geodectic Latitude measured in degrees positive from equator
% long Longitude measured in degrees positive east from Greenwich
% givendate in [Year Month Date hour minute second] format Eg. '[2016 1 1 0 0 0]'
%
% Outputs - magnetic field strength in local tangential coordinates
% Br B in radial direction
% Bt B in theta direction
% Bp B in phi direction
% Checks to see if located at either pole to avoid singularities

if (lat>-0.00000001 && lat<0.00000001)
    lat=0.00000001;
elseif(lat<180.00000001 && lat>179.99999999)
    lat=179.99999999;
end

costheta = cos((90 - lat)*pi/180);
sintheta = sin((90 - lat)*pi/180);

 ra = 6378.137; f = 1/298.257223563; b = ra*(1 - f);
    rho = hypot(ra*sintheta, b*costheta);
    r = sqrt( h.^2 + 2*h.*rho + ...
        (ra^4*sintheta.^2 + b^4*costheta.^2) ./ rho.^2 );
    cd = (h + rho) ./ r;
    sd = (ra^2 - b^2) ./ rho .* costheta.*sintheta./r;
    oldcos = costheta;
    costheta = costheta.*cd - sintheta.*sd;
    sintheta = sintheta.*cd + oldcos.*sd;
    geoclatitude=90-acos(costheta)*180/pi;
 phi = long*pi/180;


% [X,Y,Z] = geodetic2ecef(referenceEllipsoid('earth'),lat,long,h);
% [phi,theta,r] = cart2sph(X,Y,Z);
% r=r/1000;


setdate=[2015 1 1 0 0 0];
givenjd=findjd(givendate)+simtime/86400;
setjd=findjd(setdate);
days=givenjd-setjd;

% The angles must be converted from degrees into radians
% theta=(pi/2)-theta;

a=6371.2; % Reference radius used in IGRF
% This section of the code simply reads in the g and h Schmidt
% quasi-normalized coefficients

 gm=[0;1;0;1;2;0;1;2;3;0;1;2;3;4;0;1;2;3;4;5;0;1;2;3;4;5;6;0;1;2;3;4;5;6;7;0;1;2;3;4;5;6;7;8;0;1;2;3;4;5;6;7;8;9;0;1;2;3;4;5;6;7;8;9;10;0;1;2;3;4;5;6;7;8;9;10;11;0;1;2;3;4;5;6;7;8;9;10;11;12;0;1;2;3;4;5;6;7;8;9;10;11;12;13];
 gn=[1;1;2;2;2;3;3;3;3;4;4;4;4;4;5;5;5;5;5;5;6;6;6;6;6;6;6;7;7;7;7;7;7;7;7;8;8;8;8;8;8;8;8;8;9;9;9;9;9;9;9;9;9;9;10;10;10;10;10;10;10;10;10;10;10;11;11;11;11;11;11;11;11;11;11;11;11;12;12;12;12;12;12;12;12;12;12;12;12;12;13;13;13;13;13;13;13;13;13;13;13;13;13;13];
 gsvi=[10.3000000000000;18.1000000000000;-13.0500000000000;-5.71580000000000;1.81870000000000;8.50000000000000;-16.8400000000000;-1.35550000000000;-7.98480000000000;-3.06250000000000;1.10680000000000;-35.6090000000000;8.57580000000000;-3.17990000000000;-1.57500000000000;5.08330000000000;-9.99080000000000;-0.470620000000000;3.10590000000000;2.73610000000000;-4.33120000000000;-1.89030000000000;-10.4610000000000;20.9220000000000;-6.54820000000000;0.698040000000000;1.07470000000000;8.04370000000000;-7.09390000000000;-14.4800000000000;26.6220000000000;1.23490000000000;-3.70470000000000;-1.93750000000000;0.129450000000000;10.0550000000000;0;-33.6490000000000;20.7100000000000;-5.34720000000000;5.93220000000000;0.686520000000000;-1.00270000000000;0.188010000000000;0;0;0;0;0;0;0;0;0;0;0;0;0;0;0;0;0;0;0;0;0;0;0;0;0;0;0;0;0;0;0;0;0;0;0;0;0;0;0;0;0;0;0;0;0;0;0;0;0;0;0;0;0;0;0;0;0;0;0;0];
 gvali=[-29442;-1501;-3667.60000000000;5218.50000000000;1452.10000000000;3376.80000000000;-7202.40000000000;2373.40000000000;460.110000000000;3970.80000000000;4503;471.140000000000;-700.490000000000;52.0620000000000;-1831.70000000000;3661;1478.60000000000;-663.110000000000;-349.420000000000;2.87640000000000;1010.60000000000;1279.70000000000;1086.40000000000;-1294.20000000000;-157.700000000000;30.7140000000000;-47.6230000000000;2187.90000000000;-2699.20000000000;-196.930000000000;1060.80000000000;185.230000000000;58.0400000000000;-6.78110000000000;4.40140000000000;1216.60000000000;589.880000000000;-947.790000000000;-132.540000000000;-550.770000000000;198.730000000000;80.3230000000000;-39.8590000000000;-1.25340000000000;512.790000000000;1121.20000000000;336.820000000000;-273.840000000000;39.4630000000000;-448.090000000000;-1.73980000000000;65.5420000000000;-23.5140000000000;-6.39500000000000;-342.810000000000;-1532.70000000000;21.0690000000000;82.6400000000000;-58.4350000000000;133.050000000000;-28.9240000000000;42.0910000000000;19.6380000000000;-4.77860000000000;-2.13710000000000;1067.80000000000;-699.580000000000;-940.810000000000;655.940000000000;-191.610000000000;95.0540000000000;-65.8820000000000;9.92090000000000;38.6920000000000;-1.76300000000000;1.08810000000000;2.02990000000000;-1254.40000000000;-179.410000000000;318.050000000000;779.060000000000;-389.530000000000;300.620000000000;20.8300000000000;58.5270000000000;-17.5580000000000;-10.2170000000000;1.88650000000000;-2.50330000000000;0;0;-1557.20000000000;619.010000000000;641.570000000000;-492.060000000000;695.880000000000;-90.3090000000000;213.710000000000;-14.2790000000000;20.4220000000000;2.83880000000000;5.01840000000000;-1.13550000000000;-0.167020000000000];
     
 hm=[0;1;0;1;2;0;1;2;3;0;1;2;3;4;0;1;2;3;4;5;0;1;2;3;4;5;6;0;1;2;3;4;5;6;7;0;1;2;3;4;5;6;7;8;0;1;2;3;4;5;6;7;8;9;0;1;2;3;4;5;6;7;8;9;10;0;1;2;3;4;5;6;7;8;9;10;11;0;1;2;3;4;5;6;7;8;9;10;11;12;0;1;2;3;4;5;6;7;8;9;10;11;12;13];
 hn=[1;1;2;2;2;3;3;3;3;4;4;4;4;4;5;5;5;5;5;5;6;6;6;6;6;6;6;7;7;7;7;7;7;7;7;8;8;8;8;8;8;8;8;8;9;9;9;9;9;9;9;9;9;9;10;10;10;10;10;10;10;10;10;10;10;11;11;11;11;11;11;11;11;11;11;11;11;12;12;12;12;12;12;12;12;12;12;12;12;12;13;13;13;13;13;13;13;13;13;13;13;13;13;13];
 hsvi=[0;-26.6000000000000;0;-47.4580000000000;-12.2110000000000;0;25.1070000000000;-0.774600000000000;1.42300000000000;0;-7.19420000000000;20.7400000000000;6.06580000000000;-3.84550000000000;0;6.09990000000000;13.0650000000000;-5.64750000000000;7.54300000000000;0;0;0;-31.3830000000000;-6.97400000000000;1.09140000000000;2.09410000000000;0.671690000000000;0;28.3760000000000;11.5840000000000;-4.09570000000000;-3.70470000000000;-3.70470000000000;0.242180000000000;-0.129450000000000;0;-20.1090000000000;16.8250000000000;4.14200000000000;13.3680000000000;-2.96610000000000;-2.05960000000000;0.752050000000000;0;0;0;0;0;0;0;0;0;0;0;0;0;0;0;0;0;0;0;0;0;0;0;0;0;0;0;0;0;0;0;0;0;0;0;0;0;0;0;0;0;0;0;0;0;0;0;0;0;0;0;0;0;0;0;0;0;0;0;0;0];
 hvali=[0;4797.10000000000;0;-4928.70000000000;-555.900000000000;0;-353.030000000000;474.250000000000;-425.640000000000;0;1567.80000000000;-738.410000000000;378.380000000000;-243.670000000000;0;480.880000000000;1514;-561.450000000000;35.4960000000000;70.2960000000000;0;-393.180000000000;496.150000000000;586.810000000000;-363.970000000000;16.9860000000000;42.0480000000000;0;-1918.90000000000;-564.740000000000;116.730000000000;301.310000000000;20.9930000000000;-66.3580000000000;-1.42400000000000;0;677.020000000000;-1026.30000000000;550.880000000000;-390.350000000000;240.260000000000;39.1320000000000;-22.8120000000000;1.31610000000000;0;-2751.90000000000;1173.40000000000;979.200000000000;-383.360000000000;-232.470000000000;135.700000000000;7.53350000000000;-10.3360000000000;5.11600000000000;0;778.520000000000;-84.2770000000000;760.290000000000;514.230000000000;-583.930000000000;-24.7920000000000;-84.1810000000000;-22.9110000000000;-3.18570000000000;-5.16460000000000;0;-46.6390000000000;818.100000000000;-229.580000000000;-263.470000000000;126.740000000000;-18.8240000000000;-109.130000000000;-31.8640000000000;-22.0370000000000;-5.44070000000000;-1.39200000000000;0;-986.730000000000;318.050000000000;1233.50000000000;-1071.20000000000;100.210000000000;145.810000000000;-11.7050000000000;17.5580000000000;5.10870000000000;-8.48920000000000;-0.278150000000000;0.397440000000000;0;-1557.20000000000;619.010000000000;2053;-492.060000000000;-835.050000000000;-45.1550000000000;106.860000000000;-14.2790000000000;27.2290000000000;14.1940000000000;-3.01100000000000;-1.13550000000000;-0.445390000000000];

% [gn, gm, gvali, gsvi] = textread('igrfSg_sq_normalised2015.txt','%f %f %f %f');
% [hn, hm, hvali, hsvi] = textread('igrfSh_sq_normalised2015.txt','%f %f %f %f');

% igrfSg = importfile('igrfSg_sq_normalised2015.txt', 1, 104);
% gn=igrfSg(:,1);
% gm=igrfSg(:,2);
% gvali=igrfSg(:,3);
% gsvi=igrfSg(:,4);
% 
% igrfSh = importfile('igrfSh_sq_normalised2015.txt', 1, 104);
% hn=igrfSh(:,1);
% hm=igrfSh(:,2);
% hvali=igrfSh(:,3);
% hsvi=igrfSh(:,4);

N=max(gn);
g=zeros(N,N+1);
h=zeros(N,N+1);
for x=1:length(gn)
    g(gn(x),gm(x)+1) = gvali(x) + gsvi(x)*days/365;
    h(hn(x),hm(x)+1) = hvali(x) + hsvi(x)*days/365;
end
% Initialize each of the variables
% Br B in the radial driection
% Bt B in the theta direction
% Bp B in the phi direction
% P The associated Legendre polynomial evaluated at cos(theta)
% The nomenclature for the recursive values generally follows
% the form P10 = P(n-1,m-0)
% dP The partial derivative of P with respect to theta
Br=0; Bt=0; Bp=0; P20=0; dP20=0;
P11=1; P10=P11;
dP11=0; dP10=dP11;
for m=0:N
    for n=1:N
        if m<=n
            % Calculate Legendre polynomials and derivatives recursively
            if n==m
                P2 = sintheta*P11;
                dP2 = sintheta*dP11 + costheta*P11;
                P11=P2; P10=P11; P20=0;
                dP11=dP2; dP10=dP11; dP20=0;
            elseif n==1
                  P2 = costheta*P10;
                  dP2 = costheta*dP10 - sintheta*P10;
                  P20=P10; P10=P2;
                  dP20=dP10; dP10=dP2;
            else
                K = ((n-1)^2-m^2)/((2*n-1)*(2*n-3));
                P2 = costheta*P10 - K*P20;
                dP2 = costheta*dP10 - sintheta*P10 - K*dP20;
                P20=P10; P10=P2;
                dP20=dP10; dP10=dP2;
            end
            
            % Calculate Br, Bt, and Bp
            Br = Br + (a/r)^(n+2)*(n+1)*...
                ((g(n,m+1)*cos(m*phi) + h(n,m+1)*sin(m*phi))*P2);
            Bt = Bt + (a/r)^(n+2)*...
                ((g(n,m+1)*cos(m*phi) + h(n,m+1)*sin(m*phi))*dP2);
            Bp = Bp + (a/r)^(n+2)*...
                (m*(-g(n,m+1)*sin(m*phi) + h(n,m+1)*cos(m*phi))* P2);
        end
    end
end
Bt =-Bt;
Bp= -(Bp/(sintheta));

% %NED in geocentric coordinates
% Bx = -Bt;
% By = Bp;
% Bz = -Br;
% %NED in geodectic coordinates
% Bx_old = Bx;
% Bx1 = Bx.*cd + Bz.*sd;
% By1=By;
% Bz1 = Bz.*cd - Bx_old.*sd;
end
function jd=findjd(datevec)
yr=datevec(1); mon=datevec(2); day=datevec(3); hr=datevec(4); min=datevec(5); sec=datevec(6);
        jd = 367.0 * yr  ...
             - floor( (7 * (yr + floor( (mon + 9) / 12.0) ) ) * 0.25 )   ...
             + floor( 275 * mon / 9.0 ) ...
             + day + 1721013.5  ...
             + ( (sec/60.0 + min ) / 60.0 + hr ) / 24.0;
end

    function c=hypota(a,b)
        c = sqrt(abs(a).^2 + abs(b).^2)
    end

== matlab function CompleteAttDetSim/Sun Sensor/MATLAB Function ==
  data: quat output
function quat = errorquatgen()
%This function generates a quaternion representing a rotation of given
%angle in radians around some random axis
% computing first term of quaternion
angle=normrnd(0,0.0029);

q0=cos(angle/2);
%Generatiing a random axis
a=rand;
b=rand;
c=rand;
axis=[a b c];
%normalising the generated axis
nor=norm(axis);
a=a/nor;
b=b/nor;
c=c/nor;
%computing next 3 terms of quaternoin
q1=a*sin(angle/2);
q2=b*sin(angle/2);
q3=c*sin(angle/2);
%concatenate
quat=[q0 q1 q2 q3];
end

== matlab function CompleteAttDetSim/ Sun Position/Fraction Of Day ==
  data: uthr input; fracjd output; utmin input; utsec input
function fracjd=fracjday(uthr, utmin, utsec)
fracjd=uthr / 24 + utmin / 1440 + utsec / 86400;

== matlab function CompleteAttDetSim/ Sun Position/Julian Date ==
  data: month input; wholejd output; day input; year input
function wholejd = julian (month, day, year)

wholejd=0;
% Julian date

% Input

%  month = calendar month [1 - 12]
%  day   = calendar day [1 - 31]
%  year  = calendar year [yyyy]

% Output

%  jdate = Julian date

% special notes

%  (1) calendar year must include all digits

%  (2) will report October 5, 1582 to October 14, 1582
%      as invalid calendar dates and stop

% Orbital Mechanics with Matlab

%%%%%%%%%%%%%%%%%%%%%%%%%%%%%%%%%%%

y = year;
m = month;
b = 0;
c = 0;

if (m <= 2)
   y = y - 1;
   m = m + 12;
end

if (y < 0)
   c = -.75;
end

% check for valid calendar date

if (year < 1582)
   % null
elseif (year > 1582)
   a = fix(y / 100);
   b = 2 - a + floor(a / 4);
elseif (month < 10)
   % null
elseif (month > 10)
   a = fix(y / 100);
   b = 2 - a + floor(a / 4);
elseif (day <= 4)
   % null
elseif (day > 14)
   a = fix(y / 100);
   b = 2 - a + floor(a / 4);

   
   fprintf('\n\n  this is an invalid calendar date!!\n');
   

   
   return;
end

jd = fix(365.25 * y + c) + fix(30.6001 * (m + 1));
    
wholejd = jd + day + b + 1720994.5;

== matlab function CompleteAttDetSim/ Sun Position/Sun Position ECI ==
  data: jdate input; rsun output
function rsun  = sun1 (jdate)

% solar ephemeris

% input
    
%  jdate = julian day

% output

%  rasc = right ascension of the sun (radians)
%         (0 <= rasc <= 2 pi)
%  decl = declination of the sun (radians)
%         (-pi/2 <= decl <= pi/2)
%  rsun = eci position vector of the sun (kilometers)

% note

%  coordinates are inertial, geocentric,
%  equatorial and true-of-date

% Orbital Mechanics with Matlab

%%%%%%%%%%%%%%%%%%%%%%%%%%%%%%%

atr = pi / 648000;

rsun = zeros(3, 1);

% time arguments

djd = jdate - 2451545;

t = (djd / 36525) + 1;

% fundamental arguments (radians)

gs =2.0 * pi * ((0.993126 + 0.0027377785 * djd) - fix(0.993126 + 0.0027377785 * djd));
lm = 2.0 * pi * ((0.606434 + 0.03660110129 * djd) - fix(0.606434 + 0.03660110129 * djd));
ls = 2.0 * pi * ((0.606434 + 0.03660110129 * djd) - fix(0.606434 + 0.03660110129 * djd));
g2 = 2.0 * pi * ((0.606434 + 0.03660110129 * djd) - fix(0.606434 + 0.03660110129 * djd));
g4 = 2.0 * pi * ((0.606434 + 0.03660110129 * djd) - fix(0.606434 + 0.03660110129 * djd));
g5 = 2.0 * pi * ((0.606434 + 0.03660110129 * djd) - fix(0.606434 + 0.03660110129 * djd));
rm = 2.0 * pi * ((0.606434 + 0.03660110129 * djd) - fix(0.606434 + 0.03660110129 * djd));

% geocentric, ecliptic longitude of the sun (radians)

plon = 6910 * sin(gs) + 72 * sin(2 * gs) - 17 * t * sin(gs);
plon = plon - 7 * cos(gs - g5) + 6 * sin(lm - ls) ... 
       + 5 * sin(4 * gs - 8 * g4 + 3 * g5);
plon = plon - 5 * cos(2 * (gs - g2)) - 4 * (sin(gs - g2) ... 
       - cos(4 * gs - 8 * g4 + 3 * g5));
plon = plon + 3 * (sin(2 * (gs - g2)) - sin(g5) - sin(2 * (gs - g5)));
plon = ls + atr * (plon - 17 * sin(rm));

% geocentric distance of the sun (kilometers)

rsm = 149597870.691 * (1.00014 - 0.01675 * cos(gs) - 0.00014 * cos(2 * gs));

% obliquity of the ecliptic (radians)

obliq = atr * (84428 - 47 * t + 9 * cos(rm));

% geocentric, equatorial right ascension and declination (radians)

a = sin(plon) * cos(obliq);
b = cos(plon);

epsilon = 0.0000000001;
pidiv2 = 0.5 * pi;
dontenterflag=0;
c=0;
if (abs(a) < epsilon)
    rascy = (1 - sign(b)) * pidiv2;
    dontenterflag=1;
else
    c = (2 - sign(a)) * pidiv2;
end

if ((abs(b) < epsilon)&&dontenterflag~=1)
    rascy = c;
else
    rascy = c + sign(a) * sign(b) * (abs(atan(a / b)) - pidiv2);
end
   
rasc = rascy;
decl = asin(sin(obliq) * sin(plon));

% geocentric position vector of the sun (kilometers)

rsun(1) = rsm * cos(rasc) * cos(decl);
rsun(2) = rsm * sin(rasc) * cos(decl);
rsun(3) = rsm * sin(decl);

== matlab function CompleteAttDetSim/Model Workaround/Rotate about x1 ==
  data: u input; y output
function y = fcn(u)
%#codegen

y =rotx(u);

== matlab function CompleteAttDetSim/Attitude Propagator/TRIAD ==
  data: r1 input; Attitude_Matrix output; r2 input; v1 input; v2 input
function Attitude_Matrix=Triad(r1,r2,v1,v2)
%This function generates an attitude matrix two reference and two measured
%vectors.

%Tackle Anomaly 1: when both vectors are same cross product is invalid. So,
if r1==r2
    r2(1)=r2(1)+0.0000000000000001;
end
if v1==v2
    v2(1)=v2(1)+0.0000000000000001;
end
%Calculate body tirad
t1b=v1./norm(v1);
t2b=cross(t1b,v2)./norm(cross(t1b,v2));
t3b=cross(t1b,t2b)./norm(cross(t1b,t2b));

%Calculate reference tirad
t1r=r1./norm(r1);
t2r=cross(t1r,r2)./norm(cross(t1r,r2));
t3r=cross(t1r,t2r)./norm(cross(t1r,t2r));

%Calculate attituce matrix
Attitude_Matrix= t1b*(t1r.') + t2b*(t2r.') + t3b*(t3r.');

== matlab function CompleteAttDetSim/Optimised Triad/MATLAB Function ==
  data: A1 input; Attitude_Matrix output; A2 input; sigma1 input; sigma2 input
function Attitude_Matrix=Optimised_Triad(A1,A2,sigma1,sigma2)
%This function generates an optimised Attitude matrix from the following
%two attitude matrix.
%Get A1 and A2 using Traditional Traditional TRIAD using either one as
%anchor each time.

%Apply linear estimator
Acap=((sigma2)^2/((sigma1)^2+(sigma2)^2))*A1+((sigma1)^2/((sigma1)^2+(sigma2)^2))*A2;

%Orthogonalise
Attitude_Matrix=0.5*(Acap+(inv(Acap).'));

== matlab function CompleteAttDetSim/Optimised Triad/Triad Using 1 as anchor vector ==
  data: r1 input; r2 input; v1 input; v2 input; A1 output
function A1=Triad(r1,r2,v1,v2)
%This function generates an attitude matrix two reference and two measured
%vectors.

%Tackle Anomaly 1: when both vectors are same cross product is invalid. So,
% if (r1==r2)
%     r2(1)=r2(1)+0.0000000000000001;
% end
% if (v1==v2)
%     v2(1)=v2(1)+0.0000000000000001;
% end
%Calculate body tirad
t1b=v1./norm(v1);
t2b=cross(t1b,v2)./norm(cross(t1b,v2));
t3b=cross(t1b,t2b)./norm(cross(t1b,t2b));

%Calculate reference tirad
t1r=r1./norm(r1);
t2r=cross(t1r,r2)./norm(cross(t1r,r2));
t3r=cross(t1r,t2r)./norm(cross(t1r,t2r));

%Calculate attituce matrix
A1= t1b*(t1r.') + t2b*(t2r.') + t3b*(t3r.');

== matlab function CompleteAttDetSim/Optimised Triad/Triad Using 2 as anchor vector ==
  data: r1 input; A2 output; r2 input; v1 input; v2 input
function A2=Triad(r1,r2,v1,v2)
%This function generates an attitude matrix two reference and two measured
%vectors.

%Tackle Anomaly 1: when both vectors are same cross product is invalid. So,
% if (r1==r2)
%     r2(1)=r2(1)+0.0000000000000001;
% end
% if (v1==v2)
%     v2(1)=v2(1)+0.0000000000000001;
% end
%Calculate body tirad
t1b=v1./norm(v1);
t2b=cross(t1b,v2)./norm(cross(t1b,v2));
t3b=cross(t1b,t2b)./norm(cross(t1b,t2b));

%Calculate reference tirad
t1r=r1./norm(r1);
t2r=cross(t1r,r2)./norm(cross(t1r,r2));
t3r=cross(t1r,t2r)./norm(cross(t1r,t2r));

%Calculate attituce matrix
A2= t1b*(t1r.') + t2b*(t2r.') + t3b*(t3r.');

== matlab function CompleteAttDetSim/ Magnetometer/Magnetometer Error/Add Error ==
  data: y output
function y = NoiseGenerator()
typ=0.12*1/100; %typical RSS error expressed as percenage of full scale
FS=0.8;  %Full scale
y=randn(3,1)*typ*FS;
end
